simulink model "dynamiqueI"  (R2017a)
settings: Solver=VariableStepAuto  StartTime=0.0  StopTime=10.0  RelTol=1e-3
settings Model: Creator=pc  LastModifiedBy=pc

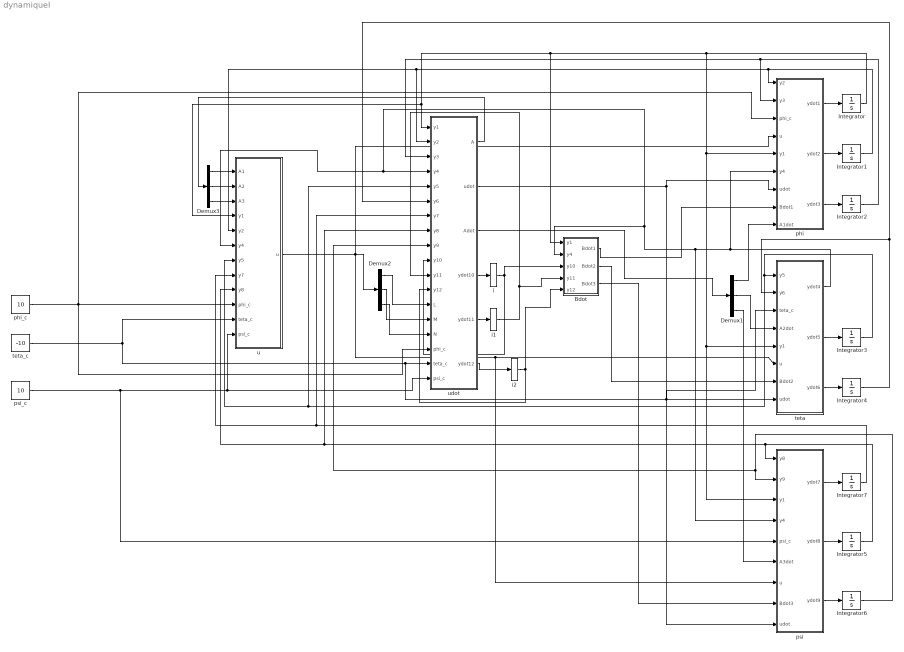
== system dynamiqueI ==
  Bdot : MATLAB Function  TreatAsAtomicUnit=on
  Demux1 : Demux  Outputs=3
  Demux2 : Demux  Outputs=3
  Demux3 : Demux  Outputs=3
  Integrator{,1..7} (8 alike) : Integrator
  i : Integrator
  i1 : Integrator
  i2 : Integrator
  phi : MATLAB Function  TreatAsAtomicUnit=on
  phi_c : Constant  Value=10
  psi : MATLAB Function  TreatAsAtomicUnit=on
  psi_c : Constant  Value=10
  teta : MATLAB Function  TreatAsAtomicUnit=on
  teta_c : Constant  Value=-10
  u : MATLAB Function  TreatAsAtomicUnit=on
  udot : MATLAB Function  TreatAsAtomicUnit=on
  wires:
  phi/1(ydot1) -> Integrator/1
  phi/2(ydot2) -> Integrator1/1
  phi/3(ydot3) -> Integrator2/1
  Integrator1/1 -> phi/1(y2), udot/2(y2), u/5(y2)
  Integrator2/1 -> phi/2(y3), udot/3(y3)
  teta/2(ydot5) -> Integrator3/1
  teta/3(ydot6) -> Integrator4/1
  Integrator3/1 -> teta/1(y5), udot/5(y5), u/7(y5)
  Integrator4/1 -> teta/2(y6), udot/6(y6)
  psi/2(ydot8) -> Integrator5/1
  psi/3(ydot9) -> Integrator6/1
  Integrator5/1 -> psi/1(y8), udot/8(y8), u/9(y8)
  Integrator6/1 -> psi/2(y9), udot/9(y9)
  teta/1(ydot4) -> phi/6(y4), psi/4(y4), Bdot/2(y4), u/6(y4), udot/4(y4)
  Integrator/1 -> phi/5(y1), psi/3(y1), teta/5(y1), Bdot/1(y1), u/4(y1), udot/1(y1)
  psi/1(ydot7) -> Integrator7/1
  udot/2(udot) -> phi/7(udot), teta/8(udot), psi/9(udot)
  udot/3(Adot) -> Demux1/1
  Demux1/1 -> phi/9(A1dot)
  Demux1/2 -> teta/4(A2dot)
  Demux1/3 -> psi/6(A3dot)
  u/1(u) -> psi/7(u), teta/6(u), Demux2/1, phi/4(u)
  Demux2/1 -> udot/13(L)
  Demux2/2 -> udot/14(M)
  Demux2/3 -> udot/15(N)
  Demux3/1 -> u/1(A1)
  Demux3/2 -> u/2(A2)
  Demux3/3 -> u/3(A3)
  udot/1(A) -> Demux3/1
  Integrator7/1 -> udot/7(y7), u/8(y7)
  phi_c/1 -> udot/16(phi_c), phi/3(phi_c), u/10(phi_c)
  teta_c/1 -> teta/3(teta_c), udot/17(teta_c), u/11(teta_c)
  psi_c/1 -> psi/5(psi_c), udot/18(psi_c), u/12(psi_c)
  udot/4(ydot10) -> i/1
  udot/5(ydot11) -> i1/1
  udot/6(ydot12) -> i2/1
  i/1 -> udot/10(y10), Bdot/3(y10)
  i1/1 -> udot/11(y11), Bdot/4(y11)
  i2/1 -> Bdot/5(y12), udot/12(y12)
  Bdot/1(Bdot1) -> phi/8(Bdot1)
  Bdot/2(Bdot2) -> teta/7(Bdot2)
  Bdot/3(Bdot3) -> psi/8(Bdot3)

== matlab function dynamiqueI/teta ==
  data: y5 input; y6 input; teta_c input; A2dot input; y1 input; u input; ydot4 output; ydot5 output; ydot6 output; Bdot2 input; udot input
function [ydot4,ydot5,ydot6] = fcn(y5,y6,teta_c,A2dot,y1,u,Bdot2,udot)
Ix=22682;
Iy=77095;
Iz=95561;
Ixz=1125;
SOM=Ix*Iz-Ixz^2;
c4=Ixz/SOM;
c7=1/Iy;
c9=Ix/SOM;
kp2=16;
phi=y1;
B2=[-c4*sind(phi),c7*cosd(phi),-c9*sind(phi)];
ydot4=y5;   
ydot5=y6+kp2*teta_c;
ydot6=A2dot+Bdot2*u+B2*udot;

== matlab function dynamiqueI/phi ==
  data: y2 input; y3 input; phi_c input; u input; y1 input; y4 input; udot input; ydot1 output; ydot2 output; ydot3 output; Bdot1 input; A1dot input
function [ydot1,ydot2,ydot3]= fcn(y2,y3,phi_c,u,y1,y4,udot,Bdot1,A1dot)
Ix=22682;
Iy=77095;
Iz=95561;
Ixz=1125;
SOM=Ix*Iz-Ixz^2;
c3=Iz/SOM;
c4=Ixz/SOM;
c7=1/Iy;
c9=Ix/SOM;
kp1=16;
phi=y1;
teta=y4;
B1=[c3+c4*cosd(phi)*tand(teta),c7*sind(phi)*tand(teta),c4+c9*cosd(phi)*tand(teta)];
%Bdot1=[c4*cosd(phi)*(tand(teta)^2 + 1)*tetadot - c4*sind(phi)*tand(teta)*phidot,c7*cosd(phi)*tand(teta)*phidot + c7*sind(phi)*(tand(teta)^2 + 1)*tetadot,c9*cosd(phi)*(tand(teta)^2 + 1)*tetadot - c9*sind(phi)*tand(teta)*phidot];
ydot1=y2;   
ydot2=y3+kp1*phi_c;
ydot3=A1dot+Bdot1*u+B1*udot;

== matlab function dynamiqueI/psi ==
  data: y8 input; y9 input; y1 input; y4 input; psi_c input; A3dot input; u input; ydot7 output; ydot8 output; ydot9 output; Bdot3 input; udot input
function [ydot7,ydot8,ydot9] = fcn(y8,y9,y1,y4,psi_c,A3dot,u,Bdot3,udot)
Ix=22682;
Iy=77095;
Iz=95561;
Ixz=1125;
SOM=Ix*Iz-Ixz^2;
c4=Ixz/SOM;
c7=1/Iy;
c9=Ix/SOM;
phi=y1;
teta=y4;
kp3=16;
ydot7=y8;
B3=[c4*cosd(phi)*(1/cosd(teta)),c7*sind(phi)*(1/cosd(teta)),c9*cosd(phi)*(1/cosd(teta))];
ydot8=y9+kp3*psi_c;
ydot9=A3dot+Bdot3*u+B3*udot;

== matlab function dynamiqueI/udot ==
  data: A output; y1 input; y2 input; y3 input; udot output; y4 input; y5 input; y6 input; y7 input; y8 input; y9 input; y10 input; y11 input; y12 input; Adot output; L input; M input; N input; ydot10 output; ydot11 output; ydot12 output; phi_c input; teta_c input; psi_c input
function [A,udot,Adot,ydot10,ydot11,ydot12]= fcn(y1,y2,y3,y4,y5,y6,y7,y8,y9,y10,y11,y12,L,M,N,phi_c,teta_c,psi_c)
kd1=6.4;kd2=6.4;kd3=6.4;
kp1=16;kp2=16;kp3=16;
Ix=22682;
Iy=77095;
Iz=95561;
Ixz=1125;
SOM=Ix*Iz-Ixz^2;
c1=((Iy-Iz)*Iz-Ixz^2)/SOM;
c2=((Ix-Iy+Iz)*Ixz)/SOM;
c3=Iz/SOM;
c4=Ixz/SOM;
c5=(Iz-Ix)/Iy;
c6=Ixz/Iy;
c7=1/Iy;
c8=(Ix*(Ix-Iy)+Ixz^2)/SOM;
c9=Ix/SOM;
%--------------------------------------------------------------------------
phi=y1;
teta=y4;
p=y10;
r=y11;
q=y12;
B=[c3+c4*cosd(phi)*tand(teta),c7*sind(phi)*tand(teta),c4+c9*cosd(phi)*tand(teta);
    -c4*sind(phi),c7*cosd(phi),-c9*sind(phi);
    c4*cosd(phi)*(1/cosd(teta)),c7*sind(phi)*(1/cosd(teta)),c9*cosd(phi)*(1/cosd(teta))];
phidot=p+tand(teta)*(q*sind(phi)+r*cosd(phi));
tetadot=q*cosd(phi)-r*sind(phi);
pp=inv(B);
A1=((c1*r+c2*p)*q)+(tetadot/cosd(teta)^2)*(q*sind(phi)+r*cosd(phi))+tand(teta)*((c5*p*r-c6*(p^2-r^2))*sind(phi)+q*(phidot*cosd(phi))+((c8*p-c2*r)*q)*cosd(phi)-r*phidot*sind(phi));
A2=(c5*p*r-c6*(p^2-r^2))*cosd(phi)-phidot*sind(phi)*q-(((c8*p-c2*r)*q)*sind(phi)+phidot*cosd(phi)*r);
A3=((c5*p*r-c6*(p^2-r^2))*sind(phi)+phidot*cosd(phi)*q+((c8*p-c2*r)*q)*cosd(phi)-phidot*sind(phi)*r)*cosd(teta)/cosd(teta)^2+(tetadot*sind(teta)*(q*sind(phi)+r*cosd(phi)))/cosd(teta)^2;
A=[A1;A2;A3];
pdot=(c1*r+c2*p)*q+c3*L+c4*N;
rdot=(c8*p-c2*r)*q+c4*L+c9*N;
qdot=c5*p*r-c6*(p^2-r^2)+c7*M;

phidotdot=pdot+(tetadot/cosd(teta)^2)*(q*sind(phi)+r*cosd(phi))+tand(teta)*(qdot*sind(phi)+q*(phidot*cosd(phi))+rdot*cosd(phi)-r*phidot*sind(phi));
tetadotdot=qdot*cosd(phi)-phidot*sind(phi)*q-(rdot*sind(phi)+phidot*cosd(phi)*r);

A1dot=(c1*rdot+c2*pdot)*q+qdot*(c1*r+c2*p)+(tetadotdot*cosd(teta)^2+2*tetadot^2*sind(teta)*cosd(teta))/cosd(teta)^4*(q*sind(phi)+r*cosd(phi))+(qdot*sind(phi)+phidot*cosd(phi)*q+rdot*cosd(phi)-phidot*sind(phi)*r)*(tetadot/cosd(teta)^2)+(tetadot/cosd(teta)^2)*((c5*p*r-c6*(p^2-r^2))*sind(phi)+q*(phidot*cosd(phi))+((c8*p-c2*r)*q)*cosd(phi)-r*phidot*sind(phi))+((c5*p*r-c6*(p^2-r^2))*phidot*cosd(phi)+(c5*(pdot*r+rdot*p)-c6*(2*p*pdot-2*r*rdot))*sind(phi)+(qdot*phidot+phidotdot*q)*cosd(phi)-phidot*sind(phi)*q*phidot+(c8*pdot-c2*rdot)*q*cosd(phi)+(qdot*cosd(phi)-phidot*sind(phi)*q)*(c8*p-c2*r)-((rdot*phidot+phidotdot*r)*sind(phi)+phidot*cosd(phi)*r*phidot))*tand(teta);
A2dot=(c5*(pdot*r+rdot*p)-c6*(2*p*pdot-2*r*rdot))*cosd(phi)-phidot*sind(phi)*(c5*p*r-c6*(p^2-r^2))-((phidotdot*q+qdot*phidot)*sind(phi)+phidot*cosd(phi)*phidot*q)-(((c8*pdot-c2*rdot)*q+qdot*(c8*p-c2*r))*sind(phi)+phidot*cosd(phi)*((c8*p-c2*r)*q)+(phidotdot*r+rdot*phidot)*cosd(phi)-phidot*sind(phi)*phidot*r);
A3dot=((((c5*(pdot*r+rdot*p)-c6*(2*p*pdot-2*r*rdot))*sind(phi)+phidot*cosd(phi)*(c5*p*r-c6*(p^2-r^2))+(phidotdot*cosd(phi)-phidot*sind(phi)*phidot)*q+qdot*phidot*cosd(phi)+((c8*pdot-c2*rdot)*q+qdot*(c8*p-c2*r))*cosd(phi)-phidot*sind(phi)*((c8*p-c2*r)*q)-((phidotdot*sind(phi)+phidot*cosd(phi)*phidot)*r+rdot*phidot*sind(phi)))*cosd(teta)-tetadot*sind(teta)*((c5*p*r-c6*(p^2-r^2))*sind(phi)+phidot*cosd(phi)*q+(c5*p*r-c6*(p^2-r^2))*cosd(phi)-phidot*sind(phi)*r))*cosd(teta)^2+2*tetadot*cosd(teta)*sind(teta)*((c5*p*r-c6*(p^2-r^2))*sind(phi)+phidot*cosd(phi)*q+((c8*p-c2*r)*q)*cosd(phi)-phidot*sind(phi)*r)*cosd(teta))/cosd(teta)^4+(((tetadotdot*sind(teta)+tetadot*cosd(teta)*tetadot)*(q*sind(phi)+r*cosd(phi))+(qdot*sind(phi)+phidot*cosd(phi)*q+rdot*cosd(phi)-phidot*sind(phi)*r)*tetadot*sind(teta))*cosd(teta)^2+2*tetadot*cosd(teta)*sind(teta)*(tetadot*sind(teta)*(q*sind(phi)+r*cosd(phi))))/cosd(teta)^4;
Adot=[A1dot;A2dot;A3dot];
ppdot=[ 0, -(c4*cosd(phi)*phidot)/(c4^2*cosd(phi)^2 + c4^2*sind(phi)^2 - c3*c9*cosd(phi)^2 - c3*c9*sind(phi)^2), (cosd(teta)*(c9*cosd(phi)^2*(tand(teta)^2 + 1)*tetadot - c4*sind(phi)*phidot + c9*sind(phi)^2*(tand(teta)^2 + 1)*tetadot))/(c4^2*cosd(phi)^2 + c4^2*sind(phi)^2 - c3*c9*cosd(phi)^2 - c3*c9*sind(phi)^2) - (sind(teta)*tetadot*(c9*tand(teta)*cosd(phi)^2 + c4*cosd(phi) + c9*tand(teta)*sind(phi)^2))/(c4^2*cosd(phi)^2 + c4^2*sind(phi)^2 - c3*c9*cosd(phi)^2 - c3*c9*sind(phi)^2);
        0,                                                    -(sind(phi)*phidot)/(c7*cosd(phi)^2 + c7*sind(phi)^2),                                                                                                                                                                                                                                                                                             (cosd(phi)*cosd(teta)*phidot)/(c7*cosd(phi)^2 + c7*sind(phi)^2) - (sind(phi)*sind(teta)*tetadot)/(c7*cosd(phi)^2 + c7*sind(phi)^2);
        0,  (c3*cosd(phi)*phidot)/(c4^2*cosd(phi)^2 + c4^2*sind(phi)^2 - c3*c9*cosd(phi)^2 - c3*c9*sind(phi)^2), (sind(teta)*tetadot*(c4*tand(teta)*cosd(phi)^2 + c3*cosd(phi) + c4*tand(teta)*sind(phi)^2))/(c4^2*cosd(phi)^2 + c4^2*sind(phi)^2 - c3*c9*cosd(phi)^2 - c3*c9*sind(phi)^2) - (cosd(teta)*(c4*cosd(phi)^2*(tand(teta)^2 + 1)*tetadot - c3*sind(phi)*phidot + c4*sind(phi)^2*(tand(teta)^2 + 1)*tetadot))/(c4^2*cosd(phi)^2 + c4^2*sind(phi)^2 - c3*c9*cosd(phi)^2 - c3*c9*sind(phi)^2)];
v=[(kp1*(phi_c-y1)-kd1*y2);(kp2*(teta_c-y4)-kd2*y5);(kp3*(psi_c-y7)-kd3*y8)];
vdot=[-kp1*y2-kd1*(y3+kp1*phi_c);-kp2*y5-kd2*(y6+kp2*teta_c);-kp3*y8-kd3*(y9+kp3*psi_c)];
udot=ppdot*(v-A)+pp*(vdot-Adot);
ydot10=(c1*r+c2*p)*q+c3*L+c4*N;  %=pdot
ydot11=(c8*p-c2*r)*q+c4*L+c9*N;  %=rdot
ydot12=c5*p*r-c6*(p^2-r^2)+c7*M; %=qdot

== matlab function dynamiqueI/u ==
  data: A1 input; A2 input; A3 input; y1 input; u output; y2 input; y4 input; y5 input; y7 input; y8 input; phi_c input; teta_c input; psi_c input
function u = fcn(A1,A2,A3,y1,y2,y4,y5,y7,y8,phi_c,teta_c,psi_c)
kd1=6.4;kd2=6.4;kd3=6.4;
kp1=16;kp2=16;kp3=16;
Ix=22682;
Iy=77095;
Iz=95561;
Ixz=1125;
SOM=Ix*Iz-Ixz^2;
c1=((Iy-Iz)*Iz-Ixz^2)/SOM;
c2=((Ix-Iy+Iz)*Ixz)/SOM;
c3=Iz/SOM;
c4=Ixz/SOM;
c5=(Iz-Ix)/Iy;
c6=Ixz/Iy;
c7=1/Iy;
c8=(Ix*(Ix-Iy)+Ixz^2)/SOM;
c9=Ix/SOM;
phi=y1;
teta=y4;
B=[c3+c4*cosd(phi)*tand(teta),c7*sind(phi)*tand(teta),c4+c9*cosd(phi)*tand(teta);
    -c4*sind(phi),c7*cosd(phi),-c9*sind(phi);
    c4*cosd(phi)*(1/cosd(teta)),c7*sind(phi)*(1/cosd(teta)),c9*cosd(phi)*(1/cosd(teta))];
pp=inv(B);
L=pp(1,:)*[(kp1*(phi_c-y1)-kd1*y2)-A1;((kp2*(teta_c-y4)-kd2*y5)-A2);((kp3*(psi_c-y7)-kd3*y8)-A3)];
M=pp(2,:)*[(kp1*(phi_c-y1)-kd1*y2)-A1;((kp2*(teta_c-y4)-kd2*y5)-A2);((kp3*(psi_c-y7)-kd3*y8)-A3)];
N=pp(3,:)*[(kp1*(phi_c-y1)-kd1*y2)-A1;((kp2*(teta_c-y4)-kd2*y5)-A2);((kp3*(psi_c-y7)-kd3*y8)-A3)];
u=[L;M;N];

== matlab function dynamiqueI/Bdot ==
  data: y1 input; Bdot1 output; y4 input; y10 input; y11 input; y12 input; Bdot2 output; Bdot3 output
function [Bdot1,Bdot2,Bdot3] = fcn(y1,y4,y10,y11,y12)
Ix=22682;
Iy=77095;
Iz=95561;
Ixz=1125;
SOM=Ix*Iz-Ixz^2;
c1=((Iy-Iz)*Iz-Ixz^2)/SOM;
c2=((Ix-Iy+Iz)*Ixz)/SOM;
c3=Iz/SOM;
c4=Ixz/SOM;
c5=(Iz-Ix)/Iy;
c6=Ixz/Iy;
c7=1/Iy;
c8=(Ix*(Ix-Iy)+Ixz^2)/SOM;
c9=Ix/SOM;
phi=y1;
teta=y4;
p=y10;
r=y11;
q=y12;
phidot=p+tand(teta)*(q*sind(phi)+r*cosd(phi));
tetadot=q*cosd(phi)-r*sind(phi);
%Bdot=[c4*cosd(phi)*(tand(teta)^2 + 1)*tetadot - c4*sind(phi)*tand(teta)*phidot,c7*cosd(phi)*tand(teta)*phidot + c7*sind(phi)*(tand(teta)^2 + 1)*tetadot,c9*cosd(phi)*(tand(teta)^2 + 1)*tetadot - c9*sind(phi)*tand(teta)*phidot;
    % -c4*cosd(phi)*phidot,-c7*sind(phi)*phidot,-c9*cosd(phi)*phidot;
     %(c4*cosd(phi)*sind(teta)*tetadot)/cosd(teta)^2 - (c4*sind(phi)*phidot)/cosd(teta), (c7*cosd(phi)*phidot)/cosd(teta) + (c7*sind(phi)*sind(teta)*tetadot)/cosd(teta)^2, (c9*cosd(phi)*sind(teta)*tetadot)/cosd(teta)^2 - (c9*sind(phi)*phidot)/cosd(teta)];
Bdot1=[c4*cosd(phi)*(tand(teta)^2 + 1)*tetadot - c4*sind(phi)*tand(teta)*phidot,c7*cosd(phi)*tand(teta)*phidot + c7*sind(phi)*(tand(teta)^2 + 1)*tetadot,c9*cosd(phi)*(tand(teta)^2 + 1)*tetadot - c9*sind(phi)*tand(teta)*phidot];
Bdot2=[ -c4*cosd(phi)*phidot,-c7*sind(phi)*phidot,-c9*cosd(phi)*phidot];
Bdot3=[(c4*cosd(phi)*sind(teta)*tetadot)/cosd(teta)^2 - (c4*sind(phi)*phidot)/cosd(teta), (c7*cosd(phi)*phidot)/cosd(teta) + (c7*sind(phi)*sind(teta)*tetadot)/cosd(teta)^2, (c9*cosd(phi)*sind(teta)*tetadot)/cosd(teta)^2 - (c9*sind(phi)*phidot)/cosd(teta)];
